simulink model "UAM_controller"  (R2024b)
settings: Solver=FixedStepAuto  StartTime=0.0  StopTime=10.0  RelTol=1e-3
undefined symbols (not defined in the file): control, controlParams, ControlSampleTime, Cruise_a, DiscIntNeverNeededParam, flightState, FWControlParams, FWTrimSpeed, uavParam, w_trim
libraries: slpidlib x41, simulink x7
(part 3 of 6)

== system UAM_controller/Auto/Multicopter Controller/Horizontal Position Control/XY Controller ==
  X_ref : Inport
  Y_ref : Inport  Port=2
  States : Inport  Port=3
  Bus Selector : BusSelector  OutputSignals=Xe,Ve,Euler
  Constant : Constant  Value=0
  Constant1 : Constant  Value=0
  Demux : Demux  Outputs=3
  Demux1 : Demux  Outputs=3
  Display{,1..10} (11 alike) : Display
  Forward position : Subsystem
  Forward position controller : slpidlib/PID Controller  Controller=PID  Form=Parallel  TimeDomain=Discrete-time  UseExternalTs=off  SampleTime=-1  IntegratorMethod=Forward Euler  FilterMethod=Forward Euler  ControllerParametersSource=internal  P=controlParams.P_X  I=controlParams.I_X  UseKiTs=off  D=controlParams.D_X  UseExternalDerivativeSource=off  N=controlParams.N_X  UseFilter=on  TunerSelectOption=Transfer Function Based (PID Tuner App)  InitialConditionSource=internal  InitialConditionForIntegrator=0  InitialConditionForFilter=0  DifferentiatorICPrevScaledInput=0  ExternalReset=none  TrackingMode=off  Kt=1  LimitOutput=off  SatLimitsSource=internal  UpperSaturationLimit=inf  LowerSaturationLimit=-inf  LinearizeAsGain=on  AntiWindupMode=none  Kb=1  LimitIntegrator=off  UpperIntegratorSaturationLimit=inf  LowerIntegratorSaturationLimit=-inf  POutMin=[]  POutMax=[]  IOutMin=[]  IOutMax=[]  DOutMin=[]  DOutMax=[]  NOutMin=[]  NOutMax=[]  SumOutMin=[]  SumOutMax=[]  SaturationOutMin=[]  SaturationOutMax=[]  PParamMin=[]  PParamMax=[]  IParamMin=[]  IParamMax=[]  DParamMin=[]  DParamMax=[]  NParamMin=[]  NParamMax=[]  KbParamMin=[]  KbParamMax=[]  KtParamMin=[]  KtParamMax=[]  KbOutMin=[]  KbOutMax=[]  KtOutMin=[]  KtOutMax=[]  IntegratorOutMin=[]  IntegratorOutMax=[]  FilterOutMin=[]  FilterOutMax=[]  SumI1OutMin=[]  SumI1OutMax=[]  SumI2OutMin=[]  SumI2OutMax=[]  SumI3OutMin=[]  SumI3OutMax=[]  SumI4OutMin=[]  SumI4OutMax=[]  SumDOutMin=[]  SumDOutMax=[]  DifferentiatorOutMin=[]  DifferentiatorOutMax=[]  FilterDiffOutCoefMin=[]  FilterDiffOutCoefMax=[]  ReciprocalOutMin=[]  ReciprocalOutMax=[]  SumDenOutMin=[]  SumDenOutMax=[]  SumNumOutMin=[]  SumNumOutMax=[]  DivideOutMin=[]  DivideOutMax=[]  UdiffTsProdOutMin=[]  UdiffTsProdOutMax=[]  NTsProdOutMin=[]  NTsProdOutMax=[]  UintegralTsProdOutMin=[]  UintegralTsProdOutMax=[]  UngainTsProdOutMin=[]  UngainTsProdOutMax=[]  ClampingZeroOutDataTypeStr=Inherit: Inherit via back propagation  ClampingZeroOutMin=[]  ClampingZeroOutMax=[]  FilterDenConstantOutDataTypeStr=Inherit: Inherit via back propagation  FilterDenConstantOutMin=[]  FilterDenConstantOutMax=[]  PCopyOutDataTypeStr=Inherit: Inherit via back propagation  PCopyOutMin=[]  PCopyOutMax=[]  NCopyOutDataTypeStr=Inherit: Inherit via back propagation  NCopyOutMin=[]  NCopyOutMax=[]  IntegratorContinuousStateAttributes=''  IntegratorStateMustResolveToSignalObject=off  IntegratorRTWStateStorageClass=Auto  FilterContinuousStateAttributes=''  FilterStateMustResolveToSignalObject=off  FilterRTWStateStorageClass=Auto  ParallelPVariant=InternalParameters  IdealPVariant=Disabled  IVariant=InternalParameters  DVariant=InternalParameters  IntegratorVariant=Discrete  SatVariant=Disabled  AWVariant=Passthrough  PCopyVariant=Disabled  TRVariant=Disabled  FdbkBlocksVariant=Forward  IdealPFdbkVariant=Disabled  SatFdbkVariant=Disabled  DerivativeFilterVariant=ForwardEulerFilter  NVariant=InternalParameters  NCopyVariant=Disabled  FilterICVariant=InternalICsFilter  IntegratorICVariant=InternalICs  ExternalResetVariant=Disabled  TRSumVariant=Passthrough  SumFdbkVariant=Disabled  SumVariant=Sum_PID  TsampFilterVariant=InternalTs  TsampNgainVariant=Passthrough  TsampIntegralVariant=Disabled_SignalSpec  ExternalSaturationOutDataTypeStr=Inherit: Same as second input  DerivativeSourceVariant=ErrorSignal  PreIntVariant=InternalPreInt
  Forward velocity : Subsystem
  Forward velocity controller : slpidlib/PID Controller  Controller=PID  Form=Parallel  TimeDomain=Discrete-time  UseExternalTs=off  SampleTime=-1  IntegratorMethod=Forward Euler  FilterMethod=Forward Euler  ControllerParametersSource=internal  P=controlParams.P_VX  I=controlParams.I_VX  UseKiTs=off  D=controlParams.D_VX  UseExternalDerivativeSource=off  N=controlParams.N_VX  UseFilter=on  TunerSelectOption=Transfer Function Based (PID Tuner App)  InitialConditionSource=internal  InitialConditionForIntegrator=0  InitialConditionForFilter=0  DifferentiatorICPrevScaledInput=0  ExternalReset=none  TrackingMode=off  Kt=1  LimitOutput=off  SatLimitsSource=internal  UpperSaturationLimit=inf  LowerSaturationLimit=-inf  LinearizeAsGain=on  AntiWindupMode=none  Kb=1  LimitIntegrator=off  UpperIntegratorSaturationLimit=inf  LowerIntegratorSaturationLimit=-inf  POutMin=[]  POutMax=[]  IOutMin=[]  IOutMax=[]  DOutMin=[]  DOutMax=[]  NOutMin=[]  NOutMax=[]  SumOutMin=[]  SumOutMax=[]  SaturationOutMin=[]  SaturationOutMax=[]  PParamMin=[]  PParamMax=[]  IParamMin=[]  IParamMax=[]  DParamMin=[]  DParamMax=[]  NParamMin=[]  NParamMax=[]  KbParamMin=[]  KbParamMax=[]  KtParamMin=[]  KtParamMax=[]  KbOutMin=[]  KbOutMax=[]  KtOutMin=[]  KtOutMax=[]  IntegratorOutMin=[]  IntegratorOutMax=[]  FilterOutMin=[]  FilterOutMax=[]  SumI1OutMin=[]  SumI1OutMax=[]  SumI2OutMin=[]  SumI2OutMax=[]  SumI3OutMin=[]  SumI3OutMax=[]  SumI4OutMin=[]  SumI4OutMax=[]  SumDOutMin=[]  SumDOutMax=[]  DifferentiatorOutMin=[]  DifferentiatorOutMax=[]  FilterDiffOutCoefMin=[]  FilterDiffOutCoefMax=[]  ReciprocalOutMin=[]  ReciprocalOutMax=[]  SumDenOutMin=[]  SumDenOutMax=[]  SumNumOutMin=[]  SumNumOutMax=[]  DivideOutMin=[]  DivideOutMax=[]  UdiffTsProdOutMin=[]  UdiffTsProdOutMax=[]  NTsProdOutMin=[]  NTsProdOutMax=[]  UintegralTsProdOutMin=[]  UintegralTsProdOutMax=[]  UngainTsProdOutMin=[]  UngainTsProdOutMax=[]  ClampingZeroOutDataTypeStr=Inherit: Inherit via back propagation  ClampingZeroOutMin=[]  ClampingZeroOutMax=[]  FilterDenConstantOutDataTypeStr=Inherit: Inherit via back propagation  FilterDenConstantOutMin=[]  FilterDenConstantOutMax=[]  PCopyOutDataTypeStr=Inherit: Inherit via back propagation  PCopyOutMin=[]  PCopyOutMax=[]  NCopyOutDataTypeStr=Inherit: Inherit via back propagation  NCopyOutMin=[]  NCopyOutMax=[]  IntegratorContinuousStateAttributes=''  IntegratorStateMustResolveToSignalObject=off  IntegratorRTWStateStorageClass=Auto  FilterContinuousStateAttributes=''  FilterStateMustResolveToSignalObject=off  FilterRTWStateStorageClass=Auto  ParallelPVariant=InternalParameters  IdealPVariant=Disabled  IVariant=InternalParameters  DVariant=InternalParameters  IntegratorVariant=Discrete  SatVariant=Disabled  AWVariant=Passthrough  PCopyVariant=Disabled  TRVariant=Disabled  FdbkBlocksVariant=Forward  IdealPFdbkVariant=Disabled  SatFdbkVariant=Disabled  DerivativeFilterVariant=ForwardEulerFilter  NVariant=InternalParameters  NCopyVariant=Disabled  FilterICVariant=InternalICsFilter  IntegratorICVariant=InternalICs  ExternalResetVariant=Disabled  TRSumVariant=Passthrough  SumFdbkVariant=Disabled  SumVariant=Sum_PID  TsampFilterVariant=InternalTs  TsampNgainVariant=Passthrough  TsampIntegralVariant=Disabled_SignalSpec  ExternalSaturationOutDataTypeStr=Inherit: Same as second input  DerivativeSourceVariant=ErrorSignal  PreIntVariant=InternalPreInt
  Lateral position : Subsystem
  Lateral position controller : slpidlib/PID Controller  Controller=PID  Form=Parallel  TimeDomain=Discrete-time  UseExternalTs=off  SampleTime=-1  IntegratorMethod=Forward Euler  FilterMethod=Forward Euler  ControllerParametersSource=internal  P=controlParams.P_Y  I=controlParams.I_Y  UseKiTs=off  D=controlParams.D_Y  UseExternalDerivativeSource=off  N=controlParams.N_Y  UseFilter=on  TunerSelectOption=Transfer Function Based (PID Tuner App)  InitialConditionSource=internal  InitialConditionForIntegrator=0  InitialConditionForFilter=0  DifferentiatorICPrevScaledInput=0  ExternalReset=none  TrackingMode=off  Kt=1  LimitOutput=off  SatLimitsSource=internal  UpperSaturationLimit=0.4  LowerSaturationLimit=-0.4  LinearizeAsGain=on  AntiWindupMode=clamping  Kb=1  LimitIntegrator=off  UpperIntegratorSaturationLimit=inf  LowerIntegratorSaturationLimit=-inf  POutMin=[]  POutMax=[]  IOutMin=[]  IOutMax=[]  DOutMin=[]  DOutMax=[]  NOutMin=[]  NOutMax=[]  SumOutMin=[]  SumOutMax=[]  SaturationOutMin=[]  SaturationOutMax=[]  PParamMin=[]  PParamMax=[]  IParamMin=[]  IParamMax=[]  DParamMin=[]  DParamMax=[]  NParamMin=[]  NParamMax=[]  KbParamMin=[]  KbParamMax=[]  KtParamMin=[]  KtParamMax=[]  KbOutMin=[]  KbOutMax=[]  KtOutMin=[]  KtOutMax=[]  IntegratorOutMin=[]  IntegratorOutMax=[]  FilterOutMin=[]  FilterOutMax=[]  SumI1OutMin=[]  SumI1OutMax=[]  SumI2OutMin=[]  SumI2OutMax=[]  SumI3OutMin=[]  SumI3OutMax=[]  SumI4OutMin=[]  SumI4OutMax=[]  SumDOutMin=[]  SumDOutMax=[]  DifferentiatorOutMin=[]  DifferentiatorOutMax=[]  FilterDiffOutCoefMin=[]  FilterDiffOutCoefMax=[]  ReciprocalOutMin=[]  ReciprocalOutMax=[]  SumDenOutMin=[]  SumDenOutMax=[]  SumNumOutMin=[]  SumNumOutMax=[]  DivideOutMin=[]  DivideOutMax=[]  UdiffTsProdOutMin=[]  UdiffTsProdOutMax=[]  NTsProdOutMin=[]  NTsProdOutMax=[]  UintegralTsProdOutMin=[]  UintegralTsProdOutMax=[]  UngainTsProdOutMin=[]  UngainTsProdOutMax=[]  ClampingZeroOutDataTypeStr=Inherit: Inherit via back propagation  ClampingZeroOutMin=[]  ClampingZeroOutMax=[]  FilterDenConstantOutDataTypeStr=Inherit: Inherit via back propagation  FilterDenConstantOutMin=[]  FilterDenConstantOutMax=[]  PCopyOutDataTypeStr=Inherit: Inherit via back propagation  PCopyOutMin=[]  PCopyOutMax=[]  NCopyOutDataTypeStr=Inherit: Inherit via back propagation  NCopyOutMin=[]  NCopyOutMax=[]  IntegratorContinuousStateAttributes=''  IntegratorStateMustResolveToSignalObject=off  IntegratorRTWStateStorageClass=Auto  FilterContinuousStateAttributes=''  FilterStateMustResolveToSignalObject=off  FilterRTWStateStorageClass=Auto  ParallelPVariant=InternalParameters  IdealPVariant=Disabled  IVariant=InternalParameters  DVariant=InternalParameters  IntegratorVariant=Discrete  SatVariant=Disabled  AWVariant=Passthrough  PCopyVariant=Disabled  TRVariant=Disabled  FdbkBlocksVariant=Forward  IdealPFdbkVariant=Disabled  SatFdbkVariant=Disabled  DerivativeFilterVariant=ForwardEulerFilter  NVariant=InternalParameters  NCopyVariant=Disabled  FilterICVariant=InternalICsFilter  IntegratorICVariant=InternalICs  ExternalResetVariant=Disabled  TRSumVariant=Passthrough  SumFdbkVariant=Disabled  SumVariant=Sum_PID  TsampFilterVariant=InternalTs  TsampNgainVariant=Passthrough  TsampIntegralVariant=Disabled_SignalSpec  ExternalSaturationOutDataTypeStr=Inherit: Same as second input  DerivativeSourceVariant=ErrorSignal  PreIntVariant=InternalPreInt
  Lateral velocity : Subsystem
  Lateral velocity controller : slpidlib/PID Controller  Controller=PID  Form=Parallel  TimeDomain=Discrete-time  UseExternalTs=off  SampleTime=-1  IntegratorMethod=Forward Euler  FilterMethod=Forward Euler  ControllerParametersSource=internal  P=controlParams.P_VY/5  I=controlParams.I_VY  UseKiTs=off  D=controlParams.D_VY  UseExternalDerivativeSource=off  N=controlParams.N_VY  UseFilter=on  TunerSelectOption=Transfer Function Based (PID Tuner App)  InitialConditionSource=internal  InitialConditionForIntegrator=0  InitialConditionForFilter=0  DifferentiatorICPrevScaledInput=0  ExternalReset=none  TrackingMode=off  Kt=1  LimitOutput=off  SatLimitsSource=internal  UpperSaturationLimit=inf  LowerSaturationLimit=-inf  LinearizeAsGain=on  AntiWindupMode=none  Kb=1  LimitIntegrator=off  UpperIntegratorSaturationLimit=inf  LowerIntegratorSaturationLimit=-inf  POutMin=[]  POutMax=[]  IOutMin=[]  IOutMax=[]  DOutMin=[]  DOutMax=[]  NOutMin=[]  NOutMax=[]  SumOutMin=[]  SumOutMax=[]  SaturationOutMin=[]  SaturationOutMax=[]  PParamMin=[]  PParamMax=[]  IParamMin=[]  IParamMax=[]  DParamMin=[]  DParamMax=[]  NParamMin=[]  NParamMax=[]  KbParamMin=[]  KbParamMax=[]  KtParamMin=[]  KtParamMax=[]  KbOutMin=[]  KbOutMax=[]  KtOutMin=[]  KtOutMax=[]  IntegratorOutMin=[]  IntegratorOutMax=[]  FilterOutMin=[]  FilterOutMax=[]  SumI1OutMin=[]  SumI1OutMax=[]  SumI2OutMin=[]  SumI2OutMax=[]  SumI3OutMin=[]  SumI3OutMax=[]  SumI4OutMin=[]  SumI4OutMax=[]  SumDOutMin=[]  SumDOutMax=[]  DifferentiatorOutMin=[]  DifferentiatorOutMax=[]  FilterDiffOutCoefMin=[]  FilterDiffOutCoefMax=[]  ReciprocalOutMin=[]  ReciprocalOutMax=[]  SumDenOutMin=[]  SumDenOutMax=[]  SumNumOutMin=[]  SumNumOutMax=[]  DivideOutMin=[]  DivideOutMax=[]  UdiffTsProdOutMin=[]  UdiffTsProdOutMax=[]  NTsProdOutMin=[]  NTsProdOutMax=[]  UintegralTsProdOutMin=[]  UintegralTsProdOutMax=[]  UngainTsProdOutMin=[]  UngainTsProdOutMax=[]  ClampingZeroOutDataTypeStr=Inherit: Inherit via back propagation  ClampingZeroOutMin=[]  ClampingZeroOutMax=[]  FilterDenConstantOutDataTypeStr=Inherit: Inherit via back propagation  FilterDenConstantOutMin=[]  FilterDenConstantOutMax=[]  PCopyOutDataTypeStr=Inherit: Inherit via back propagation  PCopyOutMin=[]  PCopyOutMax=[]  NCopyOutDataTypeStr=Inherit: Inherit via back propagation  NCopyOutMin=[]  NCopyOutMax=[]  IntegratorContinuousStateAttributes=''  IntegratorStateMustResolveToSignalObject=off  IntegratorRTWStateStorageClass=Auto  FilterContinuousStateAttributes=''  FilterStateMustResolveToSignalObject=off  FilterRTWStateStorageClass=Auto  ParallelPVariant=InternalParameters  IdealPVariant=Disabled  IVariant=InternalParameters  DVariant=InternalParameters  IntegratorVariant=Discrete  SatVariant=Disabled  AWVariant=Passthrough  PCopyVariant=Disabled  TRVariant=Disabled  FdbkBlocksVariant=Forward  IdealPFdbkVariant=Disabled  SatFdbkVariant=Disabled  DerivativeFilterVariant=ForwardEulerFilter  NVariant=InternalParameters  NCopyVariant=Disabled  FilterICVariant=InternalICsFilter  IntegratorICVariant=InternalICs  ExternalResetVariant=Disabled  TRSumVariant=Passthrough  SumFdbkVariant=Disabled  SumVariant=Sum_PID  TsampFilterVariant=InternalTs  TsampNgainVariant=Passthrough  TsampIntegralVariant=Disabled_SignalSpec  ExternalSaturationOutDataTypeStr=Inherit: Same as second input  DerivativeSourceVariant=ErrorSignal  PreIntVariant=InternalPreInt
  Selector : Selector  InputPortWidth=3  IndexOptions=Index vector (dialog)  Indices=[3]  OutputSizes=1
  SinCos : Trigonometry  Operator=sincos
  Sum{,1..5} (6 alike) : Sum  Inputs=|+-
  Terminator : Terminator
  Terminator1 : Terminator
  Forward cmd : Outport
  Sideward Cmd : Outport  Port=2
  wires:
  Demux/1 -> Sum/2
  States/1 -> Bus Selector/1
  Bus Selector/1 -> Display/1, Demux/1  "<Xe>"
  X_ref/1 -> Sum/1
  Bus Selector/2 -> Display1/1, Demux1/1  "<Ve>"
  Y_ref/1 -> Sum1/1
  Demux/2 -> Sum1/2
  Demux/3 -> Terminator/1
  Sum4/1 -> Display9/1, Forward velocity controller/1  "e_vx"
  SinCos/2 -> Forward velocity/4(cos), Lateral position/4(cos), Lateral velocity/4(cos), Forward position/4(cos)
  Selector/1 -> SinCos/1  "yaw"
  Lateral position/1(el) -> Sum2/2  "e_l"
  Sum1/1 -> Forward position/1(e_y), Lateral position/1(e_y)  "e_y"
  Sum/1 -> Forward position/2(e_x), Lateral position/2(e_x)  "e_x"
  Demux1/1 -> Forward velocity/2(vx), Lateral velocity/2(vx)
  Demux1/2 -> Forward velocity/1(vy), Lateral velocity/1(vy)
  Demux1/3 -> Terminator1/1
  SinCos/1 -> Forward velocity/3(sin), Lateral velocity/3(sin), Lateral position/3(sin), Forward position/3(sin)
  Lateral velocity/1(el) -> Sum5/2  "vl"
  Forward position/1(ef) -> Sum3/2  "e_f"
  Forward velocity/1(ef) -> Sum4/2  "vf"
  Lateral position controller/1 -> Display4/1, Sum5/1
  Forward position controller/1 -> Display8/1, Sum4/1
  Sum5/1 -> Lateral velocity controller/1, Display5/1  "e_vl"
  Bus Selector/3 -> Selector/1, Display2/1  "<Euler>"
  Constant/1 -> Sum2/1
  Sum2/1 -> Display3/1, Lateral position controller/1
  Constant1/1 -> Sum3/1
  Sum3/1 -> Forward position controller/1, Display7/1
  Lateral velocity controller/1 -> Display6/1, Sideward Cmd/1
  Forward velocity controller/1 -> Display10/1, Forward cmd/1

== system UAM_controller/Auto/Scheduler/FixedWingScheduler/Switch Case Action Subsystem ==
  note: No control allocated from fixed wing during hover.
  Action Port : ActionPort  ActionPortLabel=case [ Hover ]:
  Bus Creator : BusCreator  Inputs=4  OutDataTypeStr=Bus: FixedWingCtrlBus  NonVirtualBus=on
  Constant{,1..3} (4 alike) : Constant  Value=0
  FixedWingControls : Outport  OutDataTypeStr=Bus: FixedWingCtrlBus
  wires:
  Bus Creator/1 -> FixedWingControls/1
  Constant/1 -> Bus Creator/1  "dA"
  Constant1/1 -> Bus Creator/2  "dE"
  Constant2/1 -> Bus Creator/3  "dR"
  Constant3/1 -> Bus Creator/4  "dT"

== system UAM_controller/Auto/Scheduler/FixedWingScheduler/Switch Case Action Subsystem1 ==
  FixedWingActuators : Inport  OutDataTypeStr=Bus: FixedWingCtrlBus
  Action Port : ActionPort  ActionPortLabel=case [ Transition ]:
  Bus Creator : BusCreator  Inputs=4  OutDataTypeStr=Bus: FixedWingCtrlBus  NonVirtualBus=on
  Bus Creator1 : BusCreator  Inputs=4  OutDataTypeStr=Bus: FixedWingCtrlBus  NonVirtualBus=on
  Constant{,2..6} (6 alike) : Constant  Value=0
  Constant1 : Constant
  Demux : Demux
  FixedWingControls : Outport  OutDataTypeStr=Bus: FixedWingCtrlBus
  wires:
  Constant/1 -> Bus Creator/1  "dA"
  Constant1/1 -> Bus Creator/2  "dE"
  Constant2/1 -> Bus Creator/3  "dR"
  Constant3/1 -> Bus Creator/4  "dT"
  Demux/2 -> Bus Creator1/2  "dE"
  FixedWingActuators/1 -> Demux/1
  Bus Creator1/1 -> FixedWingControls/1
  Constant4/1 -> Bus Creator1/3  "dR"
  Constant5/1 -> Bus Creator1/4  "dT"
  Constant6/1 -> Bus Creator1/1  "dA"

== system UAM_controller/Auto/Scheduler/FixedWingScheduler/Switch Case Action Subsystem2 ==
  FixedWingActuators : Inport  OutDataTypeStr=Bus: FixedWingCtrlBus
  Action Port : ActionPort  ActionPortLabel=case [ FixedWing ]:
  Bus Creator1 : BusCreator  Inputs=4  OutDataTypeStr=Bus: FixedWingCtrlBus  NonVirtualBus=on
  Demux : Demux
  FixedWingControls : Outport  OutDataTypeStr=Bus: FixedWingCtrlBus
  wires:
  Demux/4 -> Bus Creator1/4  "dT"
  Bus Creator1/1 -> FixedWingControls/1
  Demux/3 -> Bus Creator1/3  "dR"
  Demux/2 -> Bus Creator1/2  "dE"
  FixedWingActuators/1 -> Demux/1
  Demux/1 -> Bus Creator1/1  "dA"

== system UAM_controller/Auto/Scheduler/FixedWingScheduler/Switch Case Action Subsystem3 ==
  note: No control allocated from fixed wing during hover.
  Action Port : ActionPort  ActionPortLabel=case [ BackTransition ]:
  Bus Creator : BusCreator  Inputs=4  OutDataTypeStr=Bus: FixedWingCtrlBus  NonVirtualBus=on
  Constant{,1..3} (4 alike) : Constant  Value=0
  FixedWingControls : Outport  OutDataTypeStr=Bus: FixedWingCtrlBus
  wires:
  Bus Creator/1 -> FixedWingControls/1
  Constant/1 -> Bus Creator/1  "dA"
  Constant1/1 -> Bus Creator/2  "dE"
  Constant3/1 -> Bus Creator/4  "dT"
  Constant2/1 -> Bus Creator/3  "dR"

== system UAM_controller/Auto/Scheduler/Subsystem/Actuator To Voltage ==
  Motor Commands : Inport
  Bias{,1..4} (5 alike) : Bias  Bias=1000  SaturateOnIntegerOverflow=off
  Bus Selector : BusSelector  OutputSignals=w1,w2,w3,w4,c1
  Constant : Constant  Value=0
  Display : Display
  Gain{,1..4} (5 alike) : Gain  Gain=1/(uavParam.motor.RPMMAX/360)
  Gain{5..9} (5 alike) : Gain  Gain=1000
  Saturation{,1..4} (5 alike) : Saturate  UpperLimit=2000  LowerLimit=1000
  Vector Concatenate : Concatenate  NumInputs=6
  BusElementOut : Outport  PortName=Actuator  Element=m
  wires:
  Gain6/1 -> Bias1/1
  Gain3/1 -> Gain9/1  "c1"
  Gain1/1 -> Gain7/1  "w3"
  Bus Selector/5 -> Gain3/1  "<c1>"
  Gain4/1 -> Gain6/1  "w2"
  Gain/1 -> Gain5/1  "w1"
  Motor Commands/1 -> Bus Selector/1
  Bus Selector/1 -> Gain/1  "<w1>"
  Bus Selector/4 -> Gain2/1  "<w4>"
  Gain2/1 -> Gain8/1  "w4"
  Bus Selector/3 -> Gain1/1  "<w3>"
  Bus Selector/2 -> Gain4/1  "<w2>"
  Saturation4/1 -> Vector Concatenate/5  "c1"
  Saturation2/1 -> Vector Concatenate/3  "w3"
  Saturation3/1 -> Vector Concatenate/4  "w4"
  Saturation1/1 -> Vector Concatenate/2  "w2"
  Bias3/1 -> Saturation3/1
  Saturation/1 -> Vector Concatenate/1  "w1"
  Gain8/1 -> Bias3/1
  Gain5/1 -> Bias/1
  Bias4/1 -> Saturation4/1
  Bias2/1 -> Saturation2/1
  Gain7/1 -> Bias2/1
  Bias1/1 -> Saturation1/1
  Bias/1 -> Saturation/1
  Constant/1 -> Vector Concatenate/6
  Gain9/1 -> Bias4/1
  Vector Concatenate/1 -> Display/1, BusElementOut/1

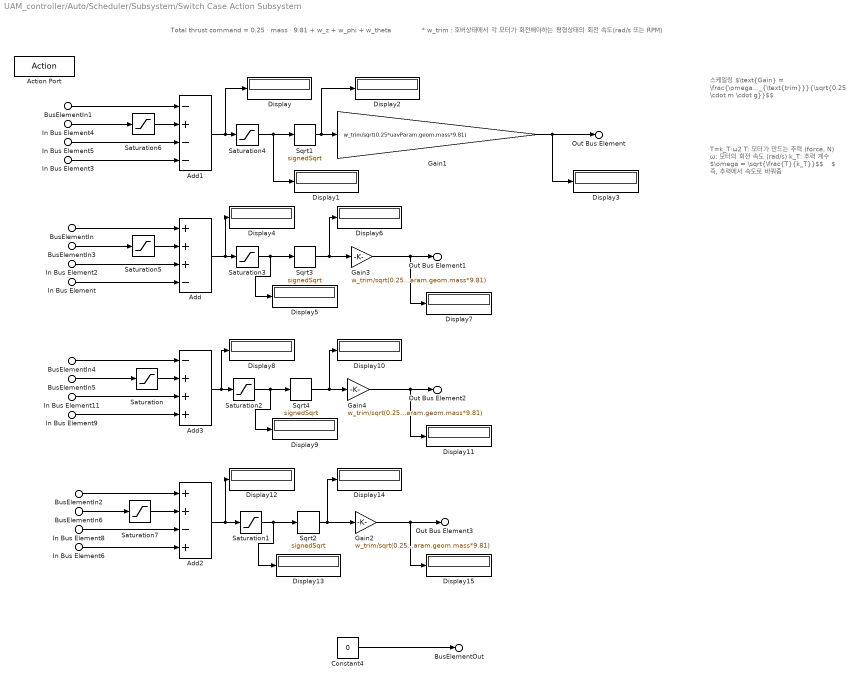
== system UAM_controller/Auto/Scheduler/Subsystem/Switch Case Action Subsystem ==
  note: * w_trim : 호버상태에서 각 모터가 회전해야하는 평형상태의 회전 속도(rad/s 또는 RPM)
  note: Total thrust command = 0.25 · mass · 9.81 + w_z + w_phi + w_theta
  note: 스케일링
      |
      | $\text{Gain} = \frac{\omega_{\text{trim}}}{\sqrt{0.25 \cdot m \cdot g}}$$
  note: T=k_T​⋅ω2
      | T: 모터가 만드는 추력 (force, N)
      | ω: 모터의 회전 속도 (rad/s)
      | k_T​: 추력 계수
      |
      | $\omega = \sqrt{\frac{T}{k_T}}$$ ​ ​ ​ ​$
      | 즉, 추력에서 속도로 바꿔줌
  In Bus Element{,3,6,9} (4 alike) : Inport  PortName=MixerCommands  Element=w_theta
  In Bus Element4 : Inport  PortName=MixerCommands  Element=w_z
  BusElementIn3 : Inport  PortName=MixerCommands  Element=w_z
  BusElementIn5 : Inport  PortName=MixerCommands  Element=w_z
  BusElementIn6 : Inport  PortName=MixerCommands  Element=w_z
  In Bus Element{2,5,8,11} (4 alike) : Inport  PortName=MixerCommands  Element=w_phi
  BusElementIn{,1..2,4} (4 alike) : Inport  PortName=MixerCommands  Element=w_psi
  Action Port : ActionPort  ActionPortLabel=case [ Hover ]:
  Add : Sum  Inputs=+++-
  Add1 : Sum  Inputs=-+--
  Add2 : Sum  Inputs=++-+
  Add3 : Sum  Inputs=-+++
  Constant4 : Constant  Value=0
  Display{,1..15} (16 alike) : Display
  Gain{1..4} (4 alike) : Gain  Gain=w_trim/sqrt(0.25*uavParam.geom.mass*9.81)
  Saturation{,1..7} (8 alike) : Saturate  UpperLimit=inf  LowerLimit=0
  Sqrt{1..4} (4 alike) : Sqrt  Operator=signedSqrt
  Out Bus Element : Outport  PortName=Actuator  Element=w1
  Out Bus Element1 : Outport  PortName=Actuator  Element=w2
  Out Bus Element2 : Outport  PortName=Actuator  Element=w3
  Out Bus Element3 : Outport  PortName=Actuator  Element=w4
  BusElementOut : Outport  PortName=Actuator  Element=c1
  wires:
  Constant4/1 -> BusElementOut/1
  In Bus Element4/1 -> Saturation6/1
  BusElementIn3/1 -> Saturation5/1
  BusElementIn5/1 -> Saturation/1
  BusElementIn6/1 -> Saturation7/1
  Add/1 -> Display4/1, Saturation3/1
  Saturation3/1 -> Display5/1, Sqrt3/1
  Sqrt3/1 -> Display6/1, Gain3/1
  Gain3/1 -> Display7/1, Out Bus Element1/1
  Add1/1 -> Display/1, Saturation4/1
  Saturation4/1 -> Display1/1, Sqrt1/1
  Sqrt1/1 -> Display2/1, Gain1/1
  Gain1/1 -> Display3/1, Out Bus Element/1
  Saturation/1 -> Add3/2
  Saturation5/1 -> Add/2
  Saturation6/1 -> Add1/2
  Saturation7/1 -> Add2/2
  BusElementIn/1 -> Add/1
  In Bus Element2/1 -> Add/3
  In Bus Element11/1 -> Add3/3
  In Bus Element9/1 -> Add3/4
  BusElementIn2/1 -> Add2/1
  In Bus Element6/1 -> Add2/4
  BusElementIn1/1 -> Add1/1
  In Bus Element5/1 -> Add1/3
  In Bus Element3/1 -> Add1/4
  In Bus Element/1 -> Add/4
  BusElementIn4/1 -> Add3/1
  In Bus Element8/1 -> Add2/3
  Add3/1 -> Display8/1, Saturation2/1
  Gain4/1 -> Display11/1, Out Bus Element2/1
  Sqrt4/1 -> Display10/1, Gain4/1
  Saturation2/1 -> Display9/1, Sqrt4/1
  Add2/1 -> Display12/1, Saturation1/1
  Gain2/1 -> Display15/1, Out Bus Element3/1
  Sqrt2/1 -> Gain2/1, Display14/1
  Saturation1/1 -> Display13/1, Sqrt2/1

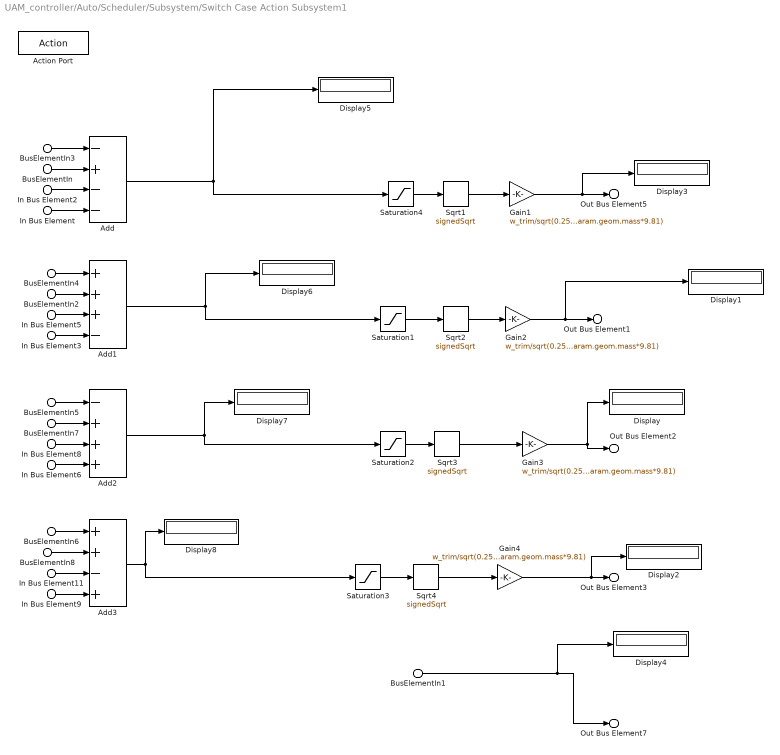
== system UAM_controller/Auto/Scheduler/Subsystem/Switch Case Action Subsystem1 ==
  In Bus Element{,3,6,9} (4 alike) : Inport  PortName=MixerCommands  Element=w_theta
  BusElementIn{,2,7..8} (4 alike) : Inport  PortName=MixerCommands  Element=w_z
  In Bus Element{2,5,8,11} (4 alike) : Inport  PortName=MixerCommands  Element=w_phi
  BusElementIn{3..6} (4 alike) : Inport  PortName=MixerCommands  Element=w_psi
  BusElementIn1 : Inport  PortName=MixerCommands  Element=cruise
  Action Port : ActionPort  ActionPortLabel=case [ Transition ]:
  Add : Sum  Inputs=-+--
  Add1 : Sum  Inputs=+++-
  Add2 : Sum  Inputs=-+++
  Add3 : Sum  Inputs=++-+
  Display{,1..8} (9 alike) : Display
  Gain{1..4} (4 alike) : Gain  Gain=w_trim/sqrt(0.25*uavParam.geom.mass*9.81)
  Saturation{1..4} (4 alike) : Saturate  UpperLimit=inf  LowerLimit=0
  Sqrt{1..4} (4 alike) : Sqrt  Operator=signedSqrt
  Out Bus Element5 : Outport  PortName=Actuator  Element=w1
  Out Bus Element1 : Outport  PortName=Actuator  Element=w2
  Out Bus Element2 : Outport  PortName=Actuator  Element=w3
  Out Bus Element3 : Outport  PortName=Actuator  Element=w4
  Out Bus Element7 : Outport  PortName=Actuator  Element=c1
  wires:
  In Bus Element9/1 -> Add3/4
  In Bus Element6/1 -> Add2/4
  In Bus Element8/1 -> Add2/3
  In Bus Element/1 -> Add/4
  In Bus Element11/1 -> Add3/3
  In Bus Element3/1 -> Add1/4
  In Bus Element2/1 -> Add/3
  In Bus Element5/1 -> Add1/3
  BusElementIn/1 -> Add/2
  BusElementIn7/1 -> Add2/2
  BusElementIn8/1 -> Add3/2
  BusElementIn6/1 -> Add3/1
  BusElementIn5/1 -> Add2/1
  BusElementIn4/1 -> Add1/1
  BusElementIn3/1 -> Add/1
  Add/1 -> Saturation4/1, Display5/1
  Add1/1 -> Saturation1/1, Display6/1
  Add2/1 -> Display7/1, Saturation2/1
  Add3/1 -> Saturation3/1, Display8/1
  Sqrt1/1 -> Gain1/1
  Saturation4/1 -> Sqrt1/1
  Gain1/1 -> Display3/1, Out Bus Element5/1
  Sqrt2/1 -> Gain2/1
  Saturation1/1 -> Sqrt2/1
  Gain2/1 -> Display1/1, Out Bus Element1/1
  Sqrt3/1 -> Gain3/1
  Saturation2/1 -> Sqrt3/1
  Gain3/1 -> Out Bus Element2/1, Display/1
  Sqrt4/1 -> Gain4/1
  Saturation3/1 -> Sqrt4/1
  Gain4/1 -> Display2/1, Out Bus Element3/1
  BusElementIn2/1 -> Add1/2
  BusElementIn1/1 -> Display4/1, Out Bus Element7/1

== system UAM_controller/Auto/Scheduler/Subsystem/Switch Case Action Subsystem2 ==
  BusElementIn : Inport  PortName=FixedWingCtrlBus  Element=dT
  Action Port : ActionPort  ActionPortLabel=case [ FixedWing ]:
  Add2 : Sum
  Constant{,2..4} (4 alike) : Constant  Value=0
  Constant1 : Constant  Value=FWTrimSpeed
  Saturation2 : Saturate  UpperLimit=Inf  LowerLimit=0
  Out Bus Element : Outport  PortName=Actuator  Element=w1
  Out Bus Element1 : Outport  PortName=Actuator  Element=w2
  Out Bus Element2 : Outport  PortName=Actuator  Element=w3
  BusElementOut : Outport  PortName=Actuator  Element=w4
  BusElementOut1 : Outport  PortName=Actuator  Element=c1
  wires:
  Constant1/1 -> Add2/1
  Saturation2/1 -> BusElementOut1/1
  Add2/1 -> Saturation2/1
  BusElementIn/1 -> Add2/2
  Constant4/1 -> BusElementOut/1
  Constant/1 -> Out Bus Element/1
  Constant3/1 -> Out Bus Element2/1
  Constant2/1 -> Out Bus Element1/1

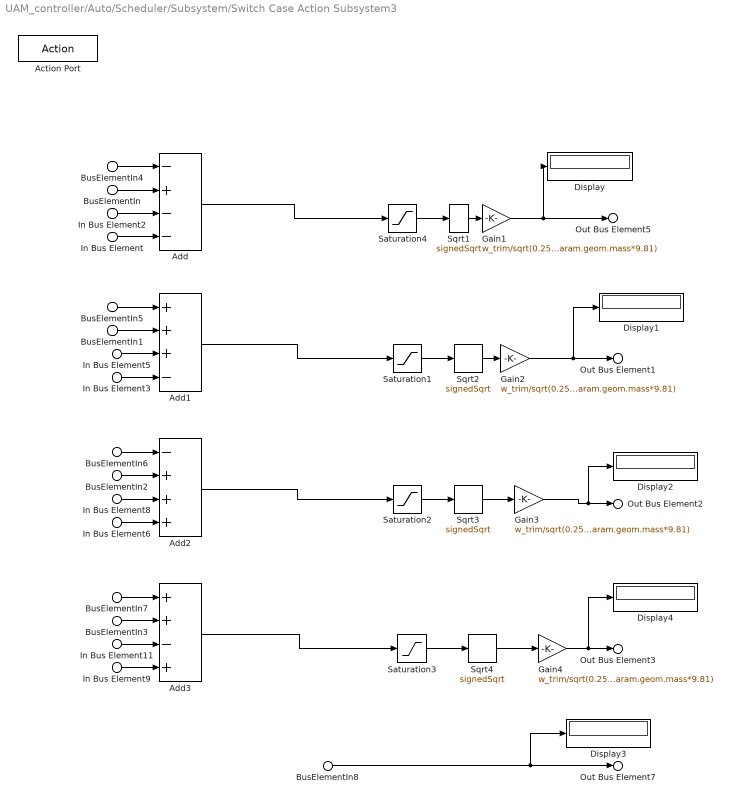
== system UAM_controller/Auto/Scheduler/Subsystem/Switch Case Action Subsystem3 ==
  In Bus Element{,3,6,9} (4 alike) : Inport  PortName=MixerCommands  Element=w_theta
  BusElementIn{,1..3} (4 alike) : Inport  PortName=MixerCommands  Element=w_z
  In Bus Element{2,5,8,11} (4 alike) : Inport  PortName=MixerCommands  Element=w_phi
  BusElementIn{4..7} (4 alike) : Inport  PortName=MixerCommands  Element=w_psi
  BusElementIn8 : Inport  PortName=MixerCommands  Element=cruise
  Action Port : ActionPort  ActionPortLabel=case [ BackTransition ]:
  Add : Sum  Inputs=-+--
  Add1 : Sum  Inputs=+++-
  Add2 : Sum  Inputs=-+++
  Add3 : Sum  Inputs=++-+
  Display{,1..4} (5 alike) : Display
  Gain{1..4} (4 alike) : Gain  Gain=w_trim/sqrt(0.25*uavParam.geom.mass*9.81)
  Saturation{1..4} (4 alike) : Saturate  UpperLimit=inf  LowerLimit=0
  Sqrt{1..4} (4 alike) : Sqrt  Operator=signedSqrt
  Out Bus Element5 : Outport  PortName=Actuator  Element=w1
  Out Bus Element1 : Outport  PortName=Actuator  Element=w2
  Out Bus Element2 : Outport  PortName=Actuator  Element=w3
  Out Bus Element3 : Outport  PortName=Actuator  Element=w4
  Out Bus Element7 : Outport  PortName=Actuator  Element=c1
  wires:
  In Bus Element9/1 -> Add3/4
  In Bus Element6/1 -> Add2/4
  In Bus Element3/1 -> Add1/4
  In Bus Element/1 -> Add/4
  In Bus Element5/1 -> Add1/3
  In Bus Element2/1 -> Add/3
  BusElementIn/1 -> Add/2
  In Bus Element11/1 -> Add3/3
  In Bus Element8/1 -> Add2/3
  BusElementIn4/1 -> Add/1
  BusElementIn5/1 -> Add1/1
  BusElementIn6/1 -> Add2/1
  BusElementIn7/1 -> Add3/1
  BusElementIn2/1 -> Add2/2
  BusElementIn3/1 -> Add3/2
  BusElementIn1/1 -> Add1/2
  BusElementIn8/1 -> Display3/1, Out Bus Element7/1
  Sqrt1/1 -> Gain1/1
  Saturation4/1 -> Sqrt1/1
  Add/1 -> Saturation4/1
  Gain1/1 -> Display/1, Out Bus Element5/1
  Sqrt2/1 -> Gain2/1
  Saturation1/1 -> Sqrt2/1
  Add1/1 -> Saturation1/1
  Gain2/1 -> Display1/1, Out Bus Element1/1
  Sqrt3/1 -> Gain3/1
  Saturation2/1 -> Sqrt3/1
  Add2/1 -> Saturation2/1
  Gain3/1 -> Display2/1, Out Bus Element2/1
  Sqrt4/1 -> Gain4/1
  Saturation3/1 -> Sqrt4/1
  Add3/1 -> Saturation3/1
  Gain4/1 -> Display4/1, Out Bus Element3/1

== system UAM_controller/Emergency/FixedWing Controller/Subsystem/Attitude Controller ==
  YPR SP : Inport
  ypr : Inport  Port=2
  Ang Rate : Inport  Port=3
  Airspeed : Inport  Port=4
  Enable : EnablePort  ShowOutputPort=on
  Compare To Constant : simulink/Logic and Bit Operations/Compare To Constant  relop===  const=uint8(1)  OutDataTypeStr=boolean
  Demux1 : Demux  Outputs=3
  Pitch Roll Controller : Subsystem
  Terminator : Terminator
  AER : Outport
  wires:
  ypr/1 -> Pitch Roll Controller/3(YPR)
  YPR SP/1 -> Demux1/1
  Enable/1 -> Compare To Constant/1
  Compare To Constant/1 -> Pitch Roll Controller/Enable
  Pitch Roll Controller/1(AER) -> AER/1
  Ang Rate/1 -> Pitch Roll Controller/4(Ang Rate)
  Airspeed/1 -> Pitch Roll Controller/5(Airspeed)
  Demux1/2 -> Pitch Roll Controller/1(Roll SP)
  Demux1/3 -> Pitch Roll Controller/2(Pitch SP)
  Demux1/1 -> Terminator/1

== system UAM_controller/Emergency/FixedWing Controller/Subsystem/Subsystem2 ==
  Euler : Inport
  pqr : Inport  Port=2
  Demux : Demux  Outputs=3
  MATLAB Function : MATLAB Function  TreatAsAtomicUnit=on
  Terminator : Terminator
  Terminator1 : Terminator
  Euler Rate : Outport
  wires:
  Demux/1 -> MATLAB Function/1(phi)
  Demux/2 -> MATLAB Function/2(theta)
  MATLAB Function/1(y) -> Terminator1/1
  pqr/1 -> Euler Rate/1
  Euler/1 -> Demux/1
  Demux/3 -> Terminator/1

== system UAM_controller/Emergency/FixedWing Controller/Subsystem/normalization ==
  In1 : Inport
  Bias : Bias  Bias=-1000  SaturateOnIntegerOverflow=off
  Gain : Gain  Gain=1/1000
  Gain1 : Gain  Gain=pi/2
  Out1 : Outport
  wires:
  Gain/1 -> Gain1/1
  In1/1 -> Bias/1
  Gain1/1 -> Out1/1
  Bias/1 -> Gain/1

== system UAM_controller/Emergency/FixedWing Controller/Subsystem/normalization1 ==
  In1 : Inport
  Bias : Bias  Bias=-1000  SaturateOnIntegerOverflow=off
  Gain : Gain  Gain=1/1000
  Gain1 : Gain  Gain=pi/6
  Out1 : Outport
  wires:
  Gain/1 -> Gain1/1
  In1/1 -> Bias/1
  Gain1/1 -> Out1/1
  Bias/1 -> Gain/1

== system UAM_controller/Emergency/FixedWing Controller/Subsystem/normalization2 ==
  In1 : Inport
  Bias : Bias  Bias=-1000  SaturateOnIntegerOverflow=off
  Gain : Gain  Gain=1/1000
  Gain1 : Gain  Gain=pi/9
  Out1 : Outport
  wires:
  Gain/1 -> Gain1/1
  In1/1 -> Bias/1
  Gain1/1 -> Out1/1
  Bias/1 -> Gain/1

== system UAM_controller/Emergency/Scheduler/FixedWingScheduler/Switch Case Action Subsystem ==
  note: No control allocated from fixed wing during hover.
  Action Port : ActionPort  ActionPortLabel=case [ Hover ]:
  Bus Creator : BusCreator  Inputs=4  OutDataTypeStr=Bus: FixedWingCtrlBus  NonVirtualBus=on
  Constant{,1..3} (4 alike) : Constant  Value=0
  FixedWingControls : Outport  OutDataTypeStr=Bus: FixedWingCtrlBus
  wires:
  Bus Creator/1 -> FixedWingControls/1
  Constant/1 -> Bus Creator/1  "dA"
  Constant1/1 -> Bus Creator/2  "dE"
  Constant2/1 -> Bus Creator/3  "dR"
  Constant3/1 -> Bus Creator/4  "dT"

== system UAM_controller/Emergency/Scheduler/FixedWingScheduler/Switch Case Action Subsystem1 ==
  FixedWingActuators : Inport  OutDataTypeStr=Bus: FixedWingCtrlBus
  TransitionDone : Inport  Port=2
  Action Port : ActionPort  ActionPortLabel=case [ Transition ]:
  Bus Creator : BusCreator  Inputs=4  OutDataTypeStr=Bus: FixedWingCtrlBus  NonVirtualBus=on
  Constant : Constant  Value=0
  Constant1 : Constant  Value=-0.2
  Constant2 : Constant  Value=0
  Constant3 : Constant  Value=0
  Switch : Switch  Criteria=u2 > Threshold  SaturateOnIntegerOverflow=off  InputSameDT=off
  FixedWingControls : Outport  OutDataTypeStr=Bus: FixedWingCtrlBus
  wires:
  Bus Creator/1 -> Switch/3
  Constant/1 -> Bus Creator/1  "dA"
  Constant1/1 -> Bus Creator/2  "dE"
  Constant2/1 -> Bus Creator/3  "dR"
  Constant3/1 -> Bus Creator/4  "dT"
  Switch/1 -> FixedWingControls/1
  TransitionDone/1 -> Switch/2

== system UAM_controller/Emergency/Scheduler/FixedWingScheduler/Switch Case Action Subsystem2 ==
  FixedWingActuators : Inport  OutDataTypeStr=Bus: FixedWingCtrlBus
  Action Port : ActionPort  ActionPortLabel=case [ FixedWing ]:
  Bus Creator : BusCreator  Inputs=4  OutDataTypeStr=Bus: FixedWingCtrlBus  NonVirtualBus=on
  Demux : Demux
  FixedWingControls : Outport  OutDataTypeStr=Bus: FixedWingCtrlBus
  wires:
  Bus Creator/1 -> FixedWingControls/1
  Demux/1 -> Bus Creator/1  "dA"
  Demux/2 -> Bus Creator/2  "dE"
  Demux/3 -> Bus Creator/3  "dR"
  Demux/4 -> Bus Creator/4  "dT"
  FixedWingActuators/1 -> Demux/1

== system UAM_controller/Emergency/Scheduler/FixedWingScheduler/Switch Case Action Subsystem3 ==
  note: No control allocated from fixed wing during hover.
  Action Port : ActionPort  ActionPortLabel=case [ BackTransition ]:
  Bus Creator : BusCreator  Inputs=4  OutDataTypeStr=Bus: FixedWingCtrlBus  NonVirtualBus=on
  Constant : Constant  Value=0
  Constant1 : Constant  Value=-0.7
  Constant2 : Constant  Value=0
  Constant3 : Constant  Value=0
  FixedWingControls : Outport  OutDataTypeStr=Bus: FixedWingCtrlBus
  wires:
  Bus Creator/1 -> FixedWingControls/1
  Constant/1 -> Bus Creator/1  "dA"
  Constant1/1 -> Bus Creator/2  "dE"
  Constant3/1 -> Bus Creator/4  "dT"
  Constant2/1 -> Bus Creator/3  "dR"

== system UAM_controller/Emergency/Scheduler/Subsystem/Actuator To Voltage ==
  Motor Commands : Inport
  Bias{,1..4} (5 alike) : Bias  Bias=1000  SaturateOnIntegerOverflow=off
  Bus Selector : BusSelector  OutputSignals=w1,w2,w3,w4,c1
  Constant : Constant  Value=0
  Gain{,1..4} (5 alike) : Gain  Gain=1/(uavParam.motor.RPMMAX/360)
  Gain{5..9} (5 alike) : Gain  Gain=1000
  Saturation{,1..4} (5 alike) : Saturate  UpperLimit=2000  LowerLimit=1000
  Vector Concatenate : Concatenate  NumInputs=6
  BusElementOut : Outport  PortName=Actuator  Element=m
  wires:
  Gain6/1 -> Bias1/1
  Gain3/1 -> Gain9/1  "c1"
  Gain1/1 -> Gain7/1  "w3"
  Bus Selector/5 -> Gain3/1  "<c1>"
  Gain4/1 -> Gain6/1  "w2"
  Gain/1 -> Gain5/1  "w1"
  Motor Commands/1 -> Bus Selector/1
  Bus Selector/1 -> Gain/1  "<w1>"
  Bus Selector/4 -> Gain2/1  "<w4>"
  Gain2/1 -> Gain8/1  "w4"
  Bus Selector/3 -> Gain1/1  "<w3>"
  Bus Selector/2 -> Gain4/1  "<w2>"
  Saturation4/1 -> Vector Concatenate/5  "c1"
  Saturation2/1 -> Vector Concatenate/3  "w3"
  Saturation3/1 -> Vector Concatenate/4  "w4"
  Saturation1/1 -> Vector Concatenate/2  "w2"
  Bias3/1 -> Saturation3/1
  Saturation/1 -> Vector Concatenate/1  "w1"
  Gain8/1 -> Bias3/1
  Gain5/1 -> Bias/1
  Bias4/1 -> Saturation4/1
  Bias2/1 -> Saturation2/1
  Gain7/1 -> Bias2/1
  Bias1/1 -> Saturation1/1
  Bias/1 -> Saturation/1
  Constant/1 -> Vector Concatenate/6
  Gain9/1 -> Bias4/1
  Vector Concatenate/1 -> BusElementOut/1

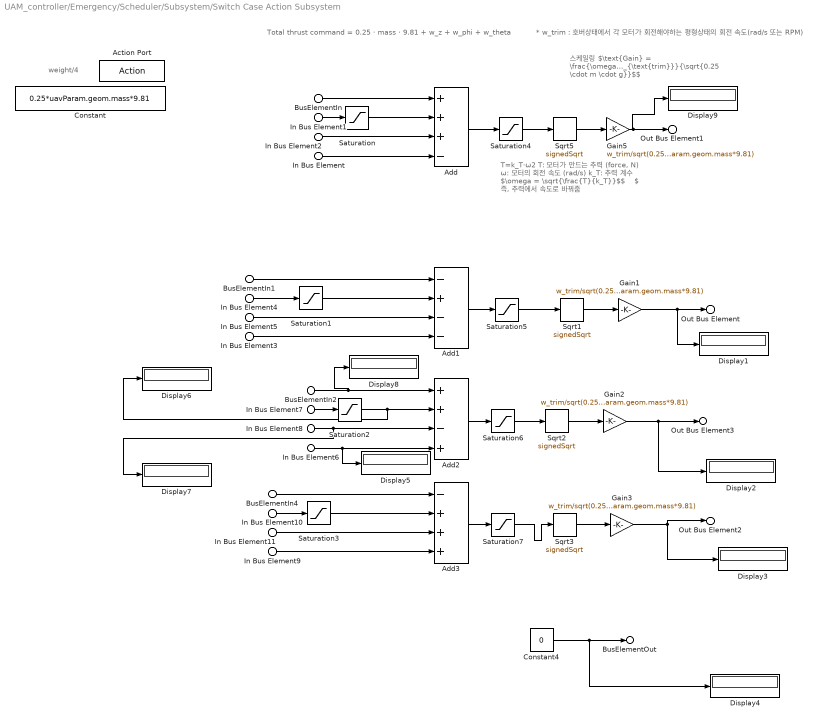
== system UAM_controller/Emergency/Scheduler/Subsystem/Switch Case Action Subsystem ==
  note: 스케일링
      |
      | $\text{Gain} = \frac{\omega_{\text{trim}}}{\sqrt{0.25 \cdot m \cdot g}}$$
  note: T=k_T​⋅ω2
      | T: 모터가 만드는 추력 (force, N)
      | ω: 모터의 회전 속도 (rad/s)
      | k_T​: 추력 계수
      |
      | $\omega = \sqrt{\frac{T}{k_T}}$$ ​ ​ ​ ​$
      | 즉, 추력에서 속도로 바꿔줌
  note: weight/4
  note: * w_trim : 호버상태에서 각 모터가 회전해야하는 평형상태의 회전 속도(rad/s 또는 RPM)
  note: Total thrust command = 0.25 · mass · 9.81 + w_z + w_phi + w_theta
  In Bus Element{,3,6,9} (4 alike) : Inport  PortName=MixerCommands  Element=w_theta
  In Bus Element{1,4,7,10} (4 alike) : Inport  PortName=MixerCommands  Element=w_z
  In Bus Element{2,5,8,11} (4 alike) : Inport  PortName=MixerCommands  Element=w_phi
  BusElementIn{,1..2,4} (4 alike) : Inport  PortName=MixerCommands  Element=w_psi
  Action Port : ActionPort  ActionPortLabel=case [ Hover ]:
  Add : Sum  Inputs=+++-
  Add1 : Sum  Inputs=-+--
  Add2 : Sum  Inputs=++-+
  Add3 : Sum  Inputs=-+++
  Constant : Constant  Value=0.25*uavParam.geom.mass*9.81
  Constant4 : Constant  Value=0
  Display{1..9} (9 alike) : Display
  Gain{1..3,5} (4 alike) : Gain  Gain=w_trim/sqrt(0.25*uavParam.geom.mass*9.81)
  Saturation{,1..3} (4 alike) : Saturate  UpperLimit=1  LowerLimit=0
  Saturation{4..7} (4 alike) : Saturate  UpperLimit=inf  LowerLimit=0
  Sqrt{1..3,5} (4 alike) : Sqrt  Operator=signedSqrt
  Out Bus Element : Outport  PortName=Actuator  Element=w1
  Out Bus Element1 : Outport  PortName=Actuator  Element=w2
  Out Bus Element2 : Outport  PortName=Actuator  Element=w3
  Out Bus Element3 : Outport  PortName=Actuator  Element=w4
  BusElementOut : Outport  PortName=Actuator  Element=c1
  wires:
  BusElementIn2/1 -> Display8/1, Add2/1
  BusElementIn1/1 -> Add1/1
  BusElementIn4/1 -> Add3/1
  Add/1 -> Saturation4/1
  Add1/1 -> Saturation5/1
  Add2/1 -> Saturation6/1
  Add3/1 -> Saturation7/1
  In Bus Element2/1 -> Add/3
  In Bus Element1/1 -> Saturation/1
  In Bus Element/1 -> Add/4
  In Bus Element4/1 -> Saturation1/1
  In Bus Element5/1 -> Add1/3
  In Bus Element3/1 -> Add1/4
  In Bus Element7/1 -> Saturation2/1
  In Bus Element8/1 -> Display7/1, Add2/3
  In Bus Element10/1 -> Saturation3/1
  In Bus Element11/1 -> Add3/3
  In Bus Element9/1 -> Add3/4
  In Bus Element6/1 -> Display5/1, Add2/4
  Constant4/1 -> Display4/1, BusElementOut/1
  BusElementIn/1 -> Add/1
  Saturation/1 -> Add/2
  Saturation1/1 -> Add1/2
  Saturation2/1 -> Display6/1, Add2/2
  Saturation3/1 -> Add3/2
  Sqrt1/1 -> Gain1/1
  Saturation5/1 -> Sqrt1/1
  Gain1/1 -> Display1/1, Out Bus Element/1
  Sqrt2/1 -> Gain2/1
  Saturation6/1 -> Sqrt2/1
  Gain2/1 -> Display2/1, Out Bus Element3/1
  Sqrt3/1 -> Gain3/1
  Saturation7/1 -> Sqrt3/1
  Gain3/1 -> Display3/1, Out Bus Element2/1
  Sqrt5/1 -> Gain5/1
  Saturation4/1 -> Sqrt5/1
  Gain5/1 -> Out Bus Element1/1, Display9/1

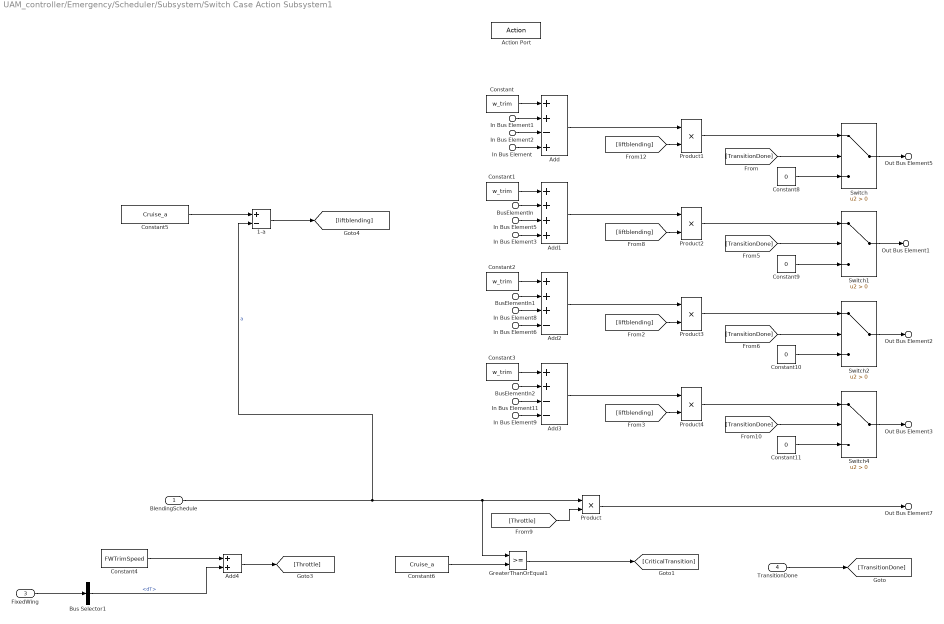
== system UAM_controller/Emergency/Scheduler/Subsystem/Switch Case Action Subsystem1 ==
  BlendingSchedule : Inport
  In Bus Element{,3,6,9} (4 alike) : Inport  Port=2  PortName=MixerCommands  Element=w_theta
  In Bus Element1 : Inport  Port=2  PortName=MixerCommands  Element=w_z
  BusElementIn : Inport  Port=2  PortName=MixerCommands  Element=w_z
  BusElementIn1 : Inport  Port=2  PortName=MixerCommands  Element=w_z
  BusElementIn2 : Inport  Port=2  PortName=MixerCommands  Element=w_z
  In Bus Element{2,5,8,11} (4 alike) : Inport  Port=2  PortName=MixerCommands  Element=w_phi
  FixedWing : Inport  Port=3
  TransitionDone : Inport  Port=4
  Action Port : ActionPort  ActionPortLabel=case [ Transition ]:
  1-a : Sum  Inputs=+-
  Add : Sum  Inputs=++-+
  Add1 : Sum  Inputs=++++
  Add2 : Sum  Inputs=+++-
  Add3 : Sum  Inputs=++--
  Add4 : Sum
  Bus Selector1 : BusSelector  OutputSignals=dT
  Constant{,1..3} (4 alike) : Constant  Value=w_trim
  Constant{8..11} (4 alike) : Constant  Value=0
  Constant4 : Constant  Value=FWTrimSpeed
  Constant5 : Constant  Value=Cruise_a
  Constant6 : Constant  Value=Cruise_a
  GreaterThanOrEqual1 : RelationalOperator  OutDataTypeStr=boolean  RndMeth=Simplest  InputSameDT=off
  Product{,1..4} (5 alike) : Product
  Switch{,1..2,4} (4 alike) : Switch  Criteria=u2 > Threshold  SaturateOnIntegerOverflow=off  InputSameDT=off
  Out Bus Element5 : Outport  PortName=Actuator  Element=w1
  Out Bus Element1 : Outport  PortName=Actuator  Element=w2
  Out Bus Element2 : Outport  PortName=Actuator  Element=w3
  Out Bus Element3 : Outport  PortName=Actuator  Element=w4
  Out Bus Element7 : Outport  PortName=Actuator  Element=c1
  wires:
  BlendingSchedule/1 -> Product/1, GreaterThanOrEqual1/1, 1-a/2  "a"
  In Bus Element9/1 -> Add3/4
  In Bus Element6/1 -> Add2/4
  In Bus Element8/1 -> Add2/3
  Constant3/1 -> Add3/1
  In Bus Element/1 -> Add/4
  Constant1/1 -> Add1/1
  In Bus Element11/1 -> Add3/3
  In Bus Element3/1 -> Add1/4
  In Bus Element2/1 -> Add/3
  Constant2/1 -> Add2/1
  In Bus Element5/1 -> Add1/3
  Constant/1 -> Add/1
  FixedWing/1 -> Bus Selector1/1
  Bus Selector1/1 -> Add4/2  "<dT>"
  Constant6/1 -> GreaterThanOrEqual1/2
  GreaterThanOrEqual1/1 -> [CriticalTransition]
  TransitionDone/1 -> [TransitionDone]
  Constant4/1 -> Add4/1
  Add4/1 -> [Throttle]
  [Throttle] -> Product/2
  Product/1 -> Out Bus Element7/1
  Constant5/1 -> 1-a/1
  In Bus Element1/1 -> Add/2
  Add/1 -> Product1/1
  1-a/1 -> [liftblending]
  [liftblending] -> Product1/2
  BusElementIn/1 -> Add1/2
  [liftblending] -> Product2/2
  Add1/1 -> Product2/1
  [liftblending] -> Product4/2
  [liftblending] -> Product3/2
  Add2/1 -> Product3/1
  Add3/1 -> Product4/1
  BusElementIn1/1 -> Add2/2
  BusElementIn2/1 -> Add3/2
  Switch/1 -> Out Bus Element5/1
  Product1/1 -> Switch/1
  [TransitionDone] -> Switch/2
  Constant8/1 -> Switch/3
  Constant9/1 -> Switch1/3
  Product2/1 -> Switch1/1
  Switch1/1 -> Out Bus Element1/1
  [TransitionDone] -> Switch1/2
  Constant10/1 -> Switch2/3
  Product3/1 -> Switch2/1
  Switch2/1 -> Out Bus Element2/1
  [TransitionDone] -> Switch2/2
  Constant11/1 -> Switch4/3
  Product4/1 -> Switch4/1
  Switch4/1 -> Out Bus Element3/1
  [TransitionDone] -> Switch4/2

== system UAM_controller/Emergency/Scheduler/Subsystem/Switch Case Action Subsystem2 ==
  BusElementIn : Inport  PortName=FixedWingCtrlBus  Element=dT
  Action Port : ActionPort  ActionPortLabel=case [ FixedWing ]:
  Add2 : Sum
  Constant{,2..4} (4 alike) : Constant  Value=0
  Constant1 : Constant  Value=FWTrimSpeed
  Saturation2 : Saturate  UpperLimit=Inf  LowerLimit=0
  Out Bus Element : Outport  PortName=Actuator  Element=w1
  Out Bus Element1 : Outport  PortName=Actuator  Element=w2
  Out Bus Element2 : Outport  PortName=Actuator  Element=w3
  BusElementOut : Outport  PortName=Actuator  Element=w4
  BusElementOut1 : Outport  PortName=Actuator  Element=c1
  wires:
  Constant1/1 -> Add2/1
  Saturation2/1 -> BusElementOut1/1
  Add2/1 -> Saturation2/1
  BusElementIn/1 -> Add2/2
  Constant4/1 -> BusElementOut/1
  Constant/1 -> Out Bus Element/1
  Constant3/1 -> Out Bus Element2/1
  Constant2/1 -> Out Bus Element1/1

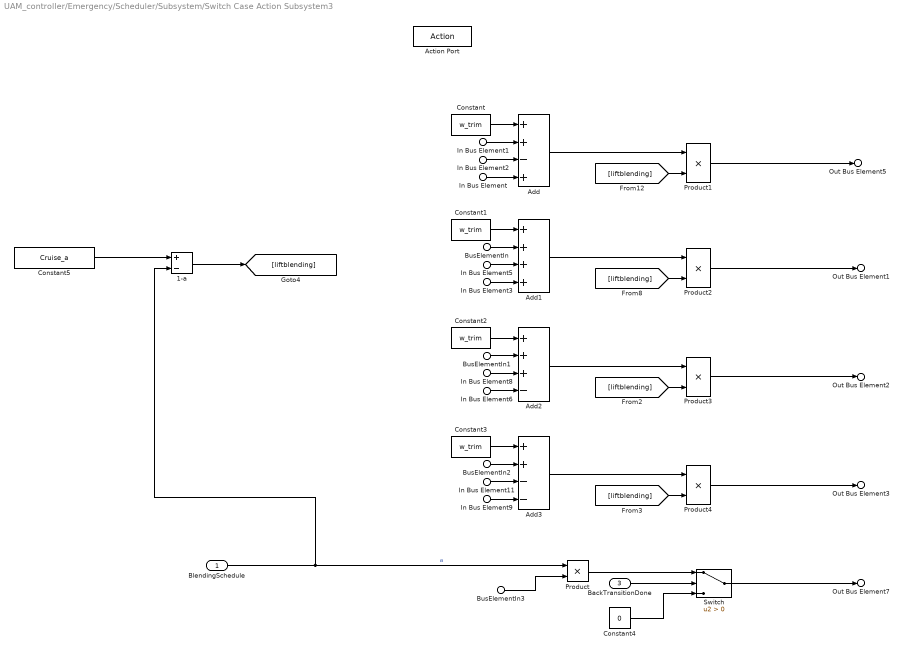
== system UAM_controller/Emergency/Scheduler/Subsystem/Switch Case Action Subsystem3 ==
  BlendingSchedule : Inport
  In Bus Element{,3,6,9} (4 alike) : Inport  Port=2  PortName=MixerCommands  Element=w_theta
  In Bus Element1 : Inport  Port=2  PortName=MixerCommands  Element=w_z
  BusElementIn : Inport  Port=2  PortName=MixerCommands  Element=w_z
  BusElementIn1 : Inport  Port=2  PortName=MixerCommands  Element=w_z
  BusElementIn2 : Inport  Port=2  PortName=MixerCommands  Element=w_z
  In Bus Element{2,5,8,11} (4 alike) : Inport  Port=2  PortName=MixerCommands  Element=w_phi
  BusElementIn3 : Inport  Port=2  PortName=MixerCommands  Element=l_x
  BackTransitionDone : Inport  Port=3
  Action Port : ActionPort  ActionPortLabel=case [ BackTransition ]:
  1-a : Sum  Inputs=+-
  Add : Sum  Inputs=++-+
  Add1 : Sum  Inputs=++++
  Add2 : Sum  Inputs=+++-
  Add3 : Sum  Inputs=++--
  Constant{,1..3} (4 alike) : Constant  Value=w_trim
  Constant4 : Constant  Value=0
  Constant5 : Constant  Value=Cruise_a
  Product{,1..4} (5 alike) : Product
  Switch : Switch  Criteria=u2 > Threshold  SaturateOnIntegerOverflow=off  InputSameDT=off
  Out Bus Element5 : Outport  PortName=Actuator  Element=w1
  Out Bus Element1 : Outport  PortName=Actuator  Element=w2
  Out Bus Element2 : Outport  PortName=Actuator  Element=w3
  Out Bus Element3 : Outport  PortName=Actuator  Element=w4
  Out Bus Element7 : Outport  PortName=Actuator  Element=c1
  wires:
  In Bus Element9/1 -> Add3/4
  1-a/1 -> [liftblending]
  In Bus Element6/1 -> Add2/4
  [liftblending] -> Product4/2
  In Bus Element3/1 -> Add1/4
  In Bus Element/1 -> Add/4
  In Bus Element5/1 -> Add1/3
  BusElementIn1/1 -> Add2/2
  Constant2/1 -> Add2/1
  BusElementIn/1 -> Add1/2
  In Bus Element2/1 -> Add/3
  [liftblending] -> Product1/2
  In Bus Element1/1 -> Add/2
  In Bus Element11/1 -> Add3/3
  BlendingSchedule/1 -> Product/1, 1-a/2  "a"
  Add/1 -> Product1/1
  [liftblending] -> Product2/2
  Constant5/1 -> 1-a/1
  In Bus Element8/1 -> Add2/3
  Constant1/1 -> Add1/1
  Add1/1 -> Product2/1
  Add3/1 -> Product4/1
  Constant3/1 -> Add3/1
  BusElementIn2/1 -> Add3/2
  Add2/1 -> Product3/1
  Constant/1 -> Add/1
  [liftblending] -> Product3/2
  Product4/1 -> Out Bus Element3/1
  Product3/1 -> Out Bus Element2/1
  Product2/1 -> Out Bus Element1/1
  Product1/1 -> Out Bus Element5/1
  BusElementIn3/1 -> Product/2
  Product/1 -> Switch/1
  Switch/1 -> Out Bus Element7/1
  Constant4/1 -> Switch/3
  BackTransitionDone/1 -> Switch/2
